simulink model "PID_Controller"  (R2020b)
settings: Solver=FixedStepAuto  StartTime=0.0  StopTime=120  RelTol=1e-3
values from neighbouring files (symbols this model uses):
  Kd = 0.0    [values.sldd]
  Ki = 49.3    [values.sldd]
  Kp = 598.0    [values.sldd]
settings Model: DataDictionary=values.sldd  Creator=shubham sharma  LastModifiedBy=shubham sharma
settings DataIOCC: SaveOutput=off  SaveTime=off

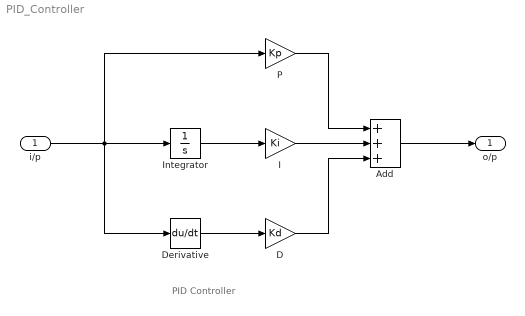
== system PID_Controller ==
  note: PID Controller
  i/p : Inport  OutDataTypeStr=double  PortDimensions=1  SampleTime=0
  Add : Sum  Inputs=+++
  D : Gain  Gain=Kd
  Derivative : Derivative
  I : Gain  Gain=Ki
  Integrator : Integrator
  P : Gain  Gain=Kp
  o/p : Outport  OutDataTypeStr=double  PortDimensions=1  SampleTime=0
  wires:
  i/p/1 -> Integrator/1, Derivative/1, P/1
  Integrator/1 -> I/1
  I/1 -> Add/2
  Derivative/1 -> D/1
  P/1 -> Add/1
  Add/1 -> o/p/1
  D/1 -> Add/3
